simulink model "Jiyeon_Project"  (R2022b)
settings: Solver=FixedStepAuto  StartTime=0.0  StopTime=inf  RelTol=1e-3  EnableMultiTasking=on
libraries: arduinolib x11, hdlsllib x1, Arduino_Additional_Lib x1, arduinosensorlib x1
settings Model: ExtModeTrigDuration=2  Creator=user  LastModifiedBy=user
settings OptimizationCC: EnhancedBackFolding=on  PassReuseOutputArgsAs=Individual arguments  ZeroExternalMemoryAtStartup=off  ZeroInternalMemoryAtStartup=off  MaxStackSize=64  OptimizeBlockOrder=speed  DifferentSizesBufferReuse=on  OptimizationCustomize=off  EfficientTunableParamExpr=on
settings DebuggingCC: ParameterTunabilityLossMsg=error
settings HardwareCC: ProdBitPerInt=16  ProdBitPerPointer=16  ProdBitPerSizeT=16  ProdBitPerPtrDiffT=16  ProdLargestAtomicFloat=None  ProdWordSize=8  ProdHWDeviceType=Atmel->AVR
settings SFSimCC: MATLABDynamicMemAlloc=off
settings RTWCC: Description=Embedded Coder  SystemTargetFile=ert.tlc  HardwareBoard=Arduino Mega 2560  TLCOptions=-aInlineSetEventsForThisBaseRateFcn=TLC_FALSE -aSuppressMultiTaskScheduler=TLC_FALSE -aRateBasedStepFcn=1  TemplateMakefile=ert_default_tmf  Toolchain=Arduino AVR  BuildConfiguration=Faster Runs
settings CodeAppCC: ForceParamTrailComments=on  IgnoreCustomStorageClasses=off  OperatorAnnotations=on  SimulinkDataObjDesc=on  SFDataObjDesc=on  InsertBlockDesc=on
settings ERTTargetCC: SupportContinuousTime=on  SupportVariableSizeSignals=on  ExtModeTransport=3  ExtModeStaticAlloc=on  ExtModeAutomaticAllocSize=off  ExtModeStaticAllocSize=2048  ExtModeMexFile=ext_xcp  ExtModeIntrfLevel=Level2 - Open

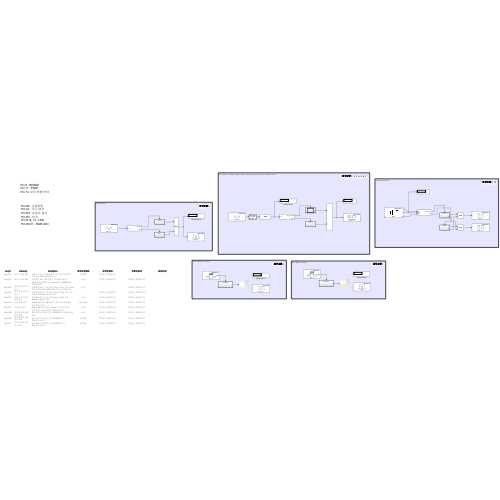
[thumbnail: Simulink's stored preview of the top-level diagram]
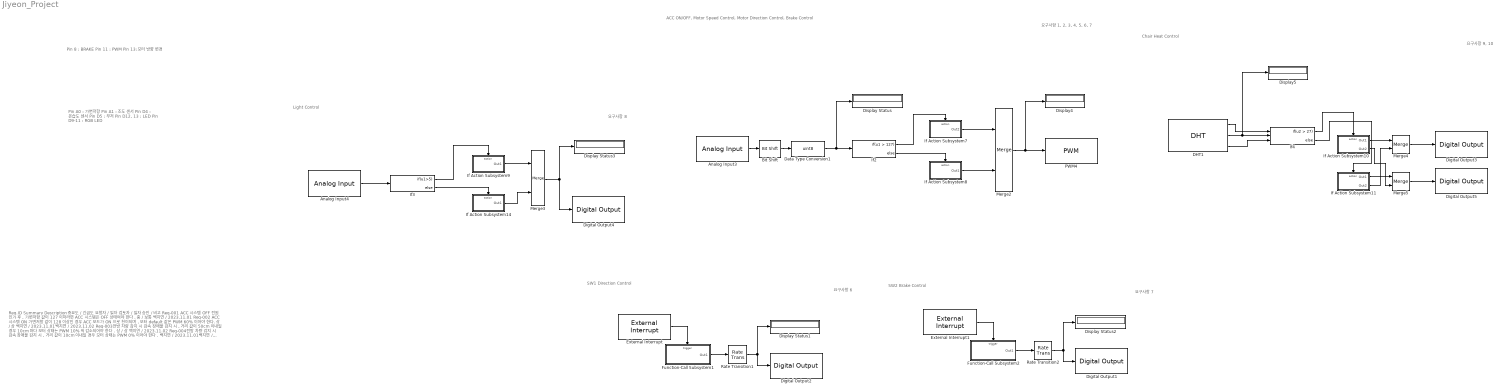
== system Jiyeon_Project ==
  note: Req.ID
      | Summary
      | Description
      | 중요도 / 긴급도
      | 요청자 / 일자
      | 검토자 / 일자
      | 승인 / 비고
      |
      | Req-001
      | ACC 시스템 OFF
      | 전원 인가 후 , 가변저항 값이 127 이하라면 ACC 시스템은 OFF 상태여야 한다 .
      | 중 / 보통
      | 백지연 / 2023.11.01
      |
      | Req-002
      | ACC 시스템 ON
      | 가변저항 값이 128 이상인 경우 ACC 모드가 ON 으로 천이되며 , 모터 default 값은 PWM 60% 이어야 한다.
      | 상 / 상
      | 백지연 / 2023.11.01
      | 백지연 / 2023.11.02
      |
      | Req-003
      | 전방 차량 감지 시 감속
      | 장애물 감지 시 , 거리 값이 50cm 이내일 경우 10cm 마다 모터 상태는 PWM 10% 씩 감소되어야 한다 .
      | 상 / 상
      |
      | 백지연 / 2023.11.02
      |
      | Req-004
      | 전방 차량 감지 시 감속
      | 장애물 감지 시 , 거리 값이 10cm 이내일 경우 모터 상태는 PWM 0% 이어야 한다 .
      |
      | 백지연 / 2023.11.01
      | 백지연 / 2023.11.02
      |
      | Req-005
      | 전방 차량 감지 시 위험 알림
      | 장애물 감지 시 , 거리 값이 30cm 이내일 경우 Buzzer 가 울려야 한다 .
      | 상 / 상
      | 백지연 / 2023.11.01
      | 백지연 / 2023.11.02
      |
      | Req-006
      | 모터 방향 변경
      | Switch 1 를 1 번 누를 때마다 , 모터의 동작 방향이 변경되어야 한다 .
      | 최상 / 최상
      | 백지연 / 2023.11.01
      | 백지연 / 2023.11.02
      |
      | Req-007
      | 브레이크 동작
      | Switch 2 를 1 번 누르면 , Brake 기능이 작동하고 다시 한번 누르면 모터가 동작해야 한다 .
      | 상 / 상
      | 백지연 / 2023.11.02
      | 백지연 / 2023.11.02
      |
      | Req-008
      | 조도에 따른 LED 자동 제어
      | 조도 값이 5 이하일 경우 , LED2( 빨강 ) 가 점등되어야 한다 .
      | 상 / 상
      | 백지연 / 2023.11.02
      | 백지연 / 2023.11.02
      |
      | Req-009
      | 온도에 따른 좌석 온도 제어
      | 온도 값이 10 이하인 경우 RGB LED R 이 점등되어야 한다 .
      | 중 / 보통
      | 백지연 / 2023.11.02
      | 백지연 / 2023.11.02
      |
      | Req-010
      | 온도에 따른 좌석 온도 제어
      | 온도 값이 10 초과인 경우 RGB LED G 가 점등되어야 한다 .
      | 중 / 보통
      | 백지연 / 2023.11.02
      | 백지연 / 2023.11.02
  note: Pin 8 : BRAKE
      | Pin 11 : PWM
      | Pin 13: 모터 방향 변경
  note: Pin A0 : 가변저항
      | Pin A1 : 조도 센서
      | Pin D4 : 온습도 센서
      | Pin D5 : 부저
      | Pin D12, 13 : LED
      | Pin D9-11 : RGB LED
  note: 요구사항 8
  note: ACC ON/OFF, Motor Speed Control, Motor Direction Control, Brake Control
  note: 요구사항 9, 10
  note: Light Control
  note: 요구사항 1, 2, 3, 4, 5, 6, 7
  note: Chair Heat Control
  note: 요구사항 6
  note: 요구사항 7
  note: SW2 Brake Control
  note: SW1 Direction Control
  Analog Input3 : arduinolib/Analog Input  pinNumber=0  ReadResultsOnly=off  ConversionTriggerSource=Software  ExternalTriggerType=uint32( 0 )  OutputDataType=uint16  EnableConversionCompleteNotify=off  EnableOuputStatus=off  SampleTime=-1  blockPlatform=arduino
  Analog Input4 : arduinolib/Analog Input  pinNumber=1  ReadResultsOnly=off  ConversionTriggerSource=Software  ExternalTriggerType=uint32( 0 )  OutputDataType=uint16  EnableConversionCompleteNotify=off  EnableOuputStatus=off  SampleTime=-1  blockPlatform=arduino
  Bit Shift : hdlsllib/Logic and Bit Operations/Bit Shift  mode=Shift Right Logical  N=3
  DHT1 : Arduino_Additional_Lib/DHT  F=off  Pin=4  Tp=11  Ts=0.5
      settings: SourceProductName=Arduino Additional Sensors Library
  Data Type Conversion1 : DataTypeConversion  OutDataTypeStr=uint8  SaturateOnIntegerOverflow=off  RndMeth=Floor
  Digital Output1 : arduinolib/Digital Output  pinNumber=8  Direction=output  blockPlatform=arduino
  Digital Output2 : arduinolib/Digital Output  pinNumber=13  Direction=output  blockPlatform=arduino
  Digital Output3 : arduinolib/Digital Output  pinNumber=9  Direction=output  blockPlatform=arduino
  Digital Output4 : arduinolib/Digital Output  pinNumber=12  Direction=output  blockPlatform=arduino
  Digital Output5 : arduinolib/Digital Output  pinNumber=10  Direction=output  blockPlatform=arduino
  Display Status{,1..3} (4 alike) : Display
  Display4 : Display
  Display5 : Display
  External Interrupt : arduinolib/External Interrupt  Pin=2  PullUp=off  Mode=FALLING  InterruptSimulationInput=off
  External Interrupt1 : arduinolib/External Interrupt  Pin=3  PullUp=off  Mode=FALLING  InterruptSimulationInput=off
  Function-Call Subsystem1 : Subsystem  TreatAsAtomicUnit=on
  Function-Call Subsystem2 : Subsystem  TreatAsAtomicUnit=on
  If Action Subsystem10 : Subsystem  TreatAsAtomicUnit=on
  If Action Subsystem11 : Subsystem  TreatAsAtomicUnit=on
  If Action Subsystem14 : Subsystem  TreatAsAtomicUnit=on
  If Action Subsystem7 : Subsystem  TreatAsAtomicUnit=on
  If Action Subsystem8 : Subsystem  TreatAsAtomicUnit=on
  If Action Subsystem9 : Subsystem  TreatAsAtomicUnit=on
  If2 : If  IfExpression=u1 > 127
  If3 : If  IfExpression=u1>5
  If4 : If  NumInputs=3  IfExpression=u2 > 27
  Merge{2..5} (4 alike) : Merge
  PWM4 : arduinolib/PWM  pinNumber=11  frequencyType=Default  desiredFrequency=490.2  achievableFrequency=490.2
  Rate Transition1 : RateTransition  Deterministic=off
  Rate Transition2 : RateTransition  Deterministic=off
  wires:
  If2/2 -> If Action Subsystem8/Action
  If2/1 -> If Action Subsystem7/Action
  If4/1 -> If Action Subsystem10/Action
  If Action Subsystem10/2(Out2) -> Merge5/2
  If Action Subsystem11/1(Out1) -> Merge5/1
  Merge5/1 -> Digital Output5/1
  DHT1/1 -> If4/1
  Analog Input3/1 -> Bit Shift/1
  Analog Input4/1 -> If3/1
  If4/2 -> If Action Subsystem11/Action
  Bit Shift/1 -> Data Type Conversion1/1
  If Action Subsystem7/1(Out2) -> Merge2/1
  Merge4/1 -> Digital Output3/1
  If Action Subsystem10/1(Out1) -> Merge4/1
  DHT1/2 -> Display5/1, If4/2
  If Action Subsystem14/1(Out1) -> Merge3/2
  Merge3/1 -> Display Status3/1, Digital Output4/1
  DHT1/3 -> If4/3
  If Action Subsystem9/1(Out1) -> Merge3/1
  Data Type Conversion1/1 -> If2/1, Display Status/1
  If Action Subsystem11/2(Out2) -> Merge4/2
  Merge2/1 -> PWM4/1, Display4/1
  If3/1 -> If Action Subsystem9/Action
  If Action Subsystem8/1(Out1) -> Merge2/2
  If3/2 -> If Action Subsystem14/Action
  Rate Transition1/1 -> Digital Output2/1, Display Status1/1
  Function-Call Subsystem2/1(Out1) -> Rate Transition2/1
  External Interrupt1/1 -> Function-Call Subsystem2/Trigger
  Rate Transition2/1 -> Digital Output1/1, Display Status2/1
  External Interrupt/1 -> Function-Call Subsystem1/Trigger
  Function-Call Subsystem1/1(Out1) -> Rate Transition1/1

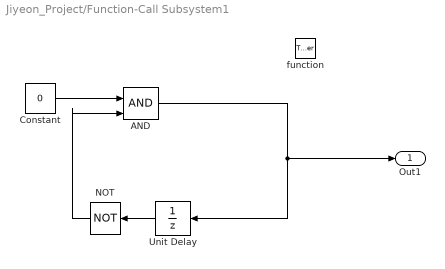
== system Jiyeon_Project/Function-Call Subsystem1 ==
  function : TriggerPort  TriggerType=function-call  VariantControl=(inherit)
  AND : Logic  IconShape=distinctive  AllPortsSameDT=off  OutDataTypeStr=boolean
  Constant : Constant  Value=0
  NOT : Logic  Operator=NOT  IconShape=distinctive  AllPortsSameDT=off  OutDataTypeStr=boolean
  Unit Delay : UnitDelay  SampleTime=-1  HasFrameUpgradeWarning=on
  Out1 : Outport
  wires:
  Constant/1 -> AND/1
  Unit Delay/1 -> NOT/1
  AND/1 -> Out1/1, Unit Delay/1
  NOT/1 -> AND/2

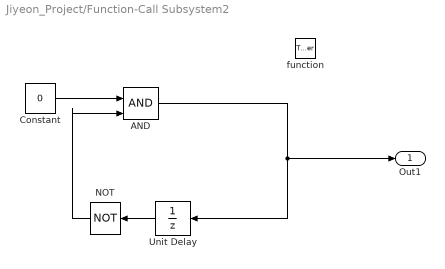
== system Jiyeon_Project/Function-Call Subsystem2 ==
  function : TriggerPort  TriggerType=function-call  VariantControl=(inherit)
  AND : Logic  IconShape=distinctive  AllPortsSameDT=off  OutDataTypeStr=boolean
  Constant : Constant  Value=0
  NOT : Logic  Operator=NOT  IconShape=distinctive  AllPortsSameDT=off  OutDataTypeStr=boolean
  Unit Delay : UnitDelay  SampleTime=-1  HasFrameUpgradeWarning=on
  Out1 : Outport
  wires:
  NOT/1 -> AND/2
  AND/1 -> Unit Delay/1, Out1/1
  Unit Delay/1 -> NOT/1
  Constant/1 -> AND/1

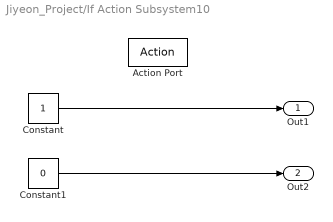
== system Jiyeon_Project/If Action Subsystem10 ==
  Action Port : ActionPort  ActionPortLabel=if(u2 > 27)
  Constant : Constant
  Constant1 : Constant  Value=0
  Out1 : Outport
  Out2 : Outport  Port=2
  wires:
  Constant/1 -> Out1/1
  Constant1/1 -> Out2/1

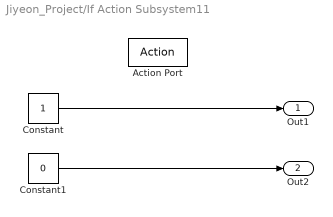
== system Jiyeon_Project/If Action Subsystem11 ==
  Action Port : ActionPort  ActionPortLabel=else
  Constant : Constant
  Constant1 : Constant  Value=0
  Out1 : Outport
  Out2 : Outport  Port=2
  wires:
  Constant/1 -> Out1/1
  Constant1/1 -> Out2/1

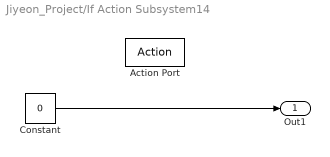
== system Jiyeon_Project/If Action Subsystem14 ==
  Action Port : ActionPort  ActionPortLabel=else
  Constant : Constant  Value=0
  Out1 : Outport
  wires:
  Constant/1 -> Out1/1

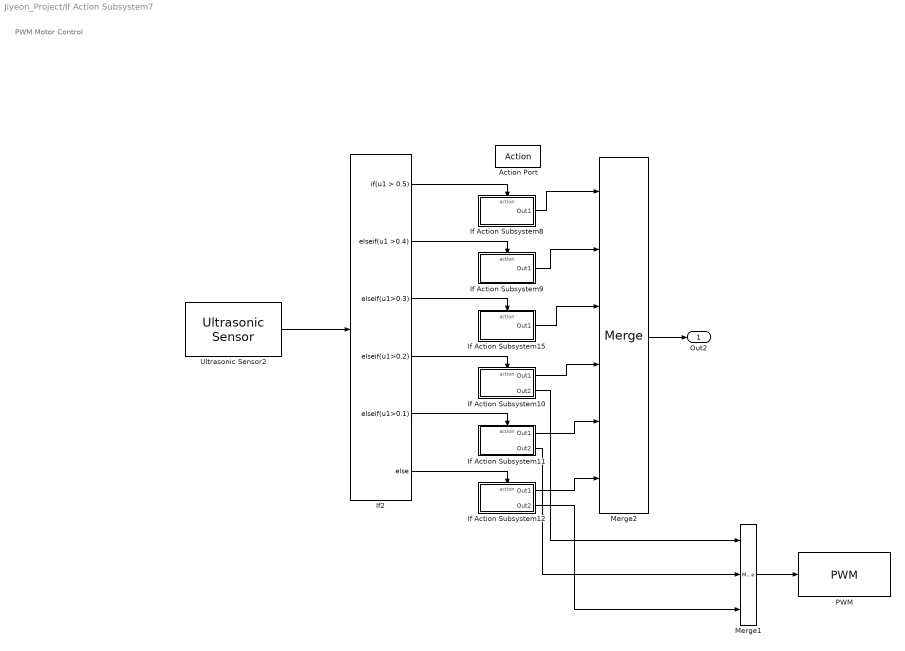
== system Jiyeon_Project/If Action Subsystem7 ==
  note: PWM Motor Control
  Action Port : ActionPort  ActionPortLabel=if(u1 > 127)
  If Action Subsystem10 : Subsystem  TreatAsAtomicUnit=on
  If Action Subsystem11 : Subsystem  TreatAsAtomicUnit=on
  If Action Subsystem12 : Subsystem  TreatAsAtomicUnit=on
  If Action Subsystem15 : Subsystem  TreatAsAtomicUnit=on
  If Action Subsystem8 : Subsystem  TreatAsAtomicUnit=on
  If Action Subsystem9 : Subsystem  TreatAsAtomicUnit=on
  If2 : If  IfExpression=u1 > 0.5  ElseIfExpressions=u1 >0.4 , u1>0.3, u1>0.2, u1>0.1
  Merge1 : Merge  Inputs=3
  Merge2 : Merge  Inputs=6
  PWM : arduinolib/PWM  pinNumber=5  frequencyType=Default  desiredFrequency=490.2  achievableFrequency=490.2
  Ultrasonic Sensor2 : arduinosensorlib/Ultrasonic Sensor  NumSignalPins=2  TrigPin=50  EchoPin=51  SignalPin=3  SampleTime_=0.1  blockPlatform=ARDUINO
  Out2 : Outport
  wires:
  If2/5 -> If Action Subsystem11/Action
  If Action Subsystem10/1(Out1) -> Merge2/4
  If Action Subsystem15/1(Out1) -> Merge2/3
  If2/4 -> If Action Subsystem10/Action
  If Action Subsystem9/1(Out1) -> Merge2/2
  If2/1 -> If Action Subsystem8/Action
  If2/3 -> If Action Subsystem15/Action
  If Action Subsystem12/1(Out1) -> Merge2/6
  If Action Subsystem8/1(Out1) -> Merge2/1
  If2/6 -> If Action Subsystem12/Action
  If Action Subsystem11/1(Out1) -> Merge2/5
  If2/2 -> If Action Subsystem9/Action
  Merge2/1 -> Out2/1
  Ultrasonic Sensor2/1 -> If2/1
  If Action Subsystem10/2(Out2) -> Merge1/1
  Merge1/1 -> PWM/1
  If Action Subsystem11/2(Out2) -> Merge1/2
  If Action Subsystem12/2(Out2) -> Merge1/3

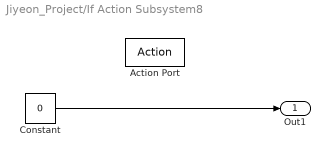
== system Jiyeon_Project/If Action Subsystem8 ==
  Action Port : ActionPort  ActionPortLabel=else
  Constant : Constant  Value=0
  Out1 : Outport
  wires:
  Constant/1 -> Out1/1

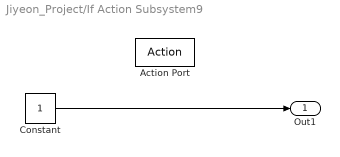
== system Jiyeon_Project/If Action Subsystem9 ==
  Action Port : ActionPort  ActionPortLabel=if(u1>5)
  Constant : Constant
  Out1 : Outport
  wires:
  Constant/1 -> Out1/1

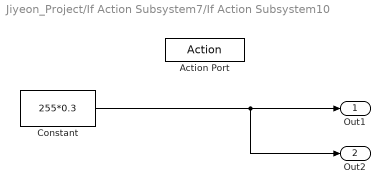
== system Jiyeon_Project/If Action Subsystem7/If Action Subsystem10 ==
  Action Port : ActionPort  ActionPortLabel=elseif( u1>0.2)
  Constant : Constant  Value=255*0.3
  Out1 : Outport
  Out2 : Outport  Port=2
  wires:
  Constant/1 -> Out1/1, Out2/1

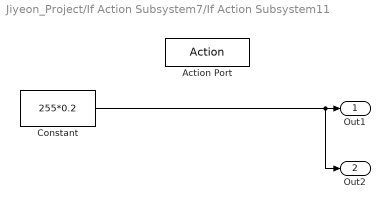
== system Jiyeon_Project/If Action Subsystem7/If Action Subsystem11 ==
  Action Port : ActionPort  ActionPortLabel=elseif( u1>0.1)
  Constant : Constant  Value=255*0.2
  Out1 : Outport
  Out2 : Outport  Port=2
  wires:
  Constant/1 -> Out2/1, Out1/1

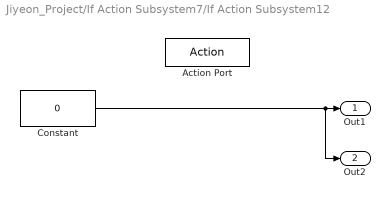
== system Jiyeon_Project/If Action Subsystem7/If Action Subsystem12 ==
  Action Port : ActionPort  ActionPortLabel=else
  Constant : Constant  Value=0
  Out1 : Outport
  Out2 : Outport  Port=2
  wires:
  Constant/1 -> Out2/1, Out1/1

== system Jiyeon_Project/If Action Subsystem7/If Action Subsystem15 ==
  Action Port : ActionPort  ActionPortLabel=elseif( u1>0.3)
  Constant : Constant  Value=255*0.4
  Out1 : Outport
  wires:
  Constant/1 -> Out1/1

== system Jiyeon_Project/If Action Subsystem7/If Action Subsystem8 ==
  Action Port : ActionPort  ActionPortLabel=if(u1 > 0.5)
  Constant : Constant  Value=255*0.6
  Out1 : Outport
  wires:
  Constant/1 -> Out1/1

== system Jiyeon_Project/If Action Subsystem7/If Action Subsystem9 ==
  Action Port : ActionPort  ActionPortLabel=elseif(u1 >0.4 )
  Constant : Constant  Value=255*0.5
  Out1 : Outport
  wires:
  Constant/1 -> Out1/1
